simulink model "ATRIAS_vnmc"  (R2015a)
settings: Solver=ode45  StartTime=0.0  StopTime=60  FixedStep=1e-3  MinStep=1e-6  RelTol=1e-3  AbsTol=1e-4
values from neighbouring files (symbols this model uses):
  initial_boom_yaw = initial_boom_yaw + delta_yaw0    [run_model.m]
  max_floor_diff = cost_fun_opts.max_floor_diff    [opt_cmaes.m]    (also in run_model.m; set_all_params_simple.m = 0)
  noise_on_off = cost_fun_opts.noise_on_off    [opt_cmaes.m]    (also in run_model.m; set_all_params_simple.m = 0)
  noise_seed = cost_fun_opts.noise_seed    [opt_cmaes.m]    (also in run_model.m; set_all_params_simple.m = 1)
  noise_variance = cost_fun_opts.noise_variance    [opt_cmaes.m]    (also in run_model.m; set_all_params_simple.m = 0.000174532925199)
  SEA_swing_ctrl_on_off = cost_fun_opts.SEA_swing_ctrl_on_off    [opt_cmaes.m]    (also in run_model.m; set_all_params_simple.m = 0)
  sim_t = simout.twalk    [run_model.m]
  steady_dist = cost_fun_opts.steady_dist    [opt_cmaes.m]    (also in run_model.m; set_all_params_simple.m = 10)
  ts_anim = 0.0333    [run_model.m]
undefined symbols (not defined in the file or in its folder): A1_notch_f1, A2_notch_f1, A_lpf_dtau, A_lpf_velocity, B1_lpf_dtau, B1_lpf_velocity, B1_notch_f1, B2_lpf_dtau, B2_lpf_velocity, B2_notch_f1, b_hmotor, b_leg_spring, b_rotor, base_color_d, boom_color_d, boom_mount_to_center_diagonal, breakaway_friction, c, c_jointstop, com_height_offset, contactThr, coulomb_friction, CtrlPar_theta0, D12_S, D12_T, d_com, ddx_max, ddy_max, delta_phi_max, delta_phi_max_buffer, delta_phi_max_dropoff, delta_phi_min, des_forward_velocity, DS_width, dtau_des_max, dtheta0_vmc, dx0_vmc, dy_max, eref, fblink_color_d, fcut_acceleration, floor_color_d, floor_tile_width, floor_zero_height, FmaxBFSH, FmaxGLU, FmaxHAM, FmaxHFL, FmaxRF, FmaxVAS, FPCtrlPar, friction_linear_zone, g, gain_nodes_sea_torque, gamma_stance_thr, gamma_swing_thr, hip_height, HIP_MTR_MAX_CONT_TORQUE, HIP_MTR_MAX_TORQUE, hshaft_color_d ... (+236)
libraries: sm_lib x280, nesl_utility x174, simulink x114, simulink_extras x58, fl_lib x16, mblibv1 x2, dspswit3 x2
(part 6 of 23)

== system ATRIAS_vnmc/atrias_system/ATRIAS Mechanical System Layer/Torso ==
  COM Sensor : Subsystem
  COM accelerations : Scope
      settings: TimeRange=3  YMin=-750  YMax=2750  SaveName=ScopeData27
  COM dx : Scope
      settings: TimeRange=4  YMin=2.85  YMax=3.95  SaveName=ScopeData24
  COM dy : Scope
      settings: TimeRange=4  YMin=-1.1  YMax=1.2  SaveName=ScopeData32
  COM y pos : Scope
      settings: TimeRange=3  YMin=0.875  YMax=1.375  SaveName=ScopeData23
  CS1 to CS2 : sm_lib/Frames and Transforms/Rigid Transform  TranslationMethod=Cartesian  TranslationLengthUnit=m  TranslationStandardAxis=+Z  TranslationStandardOffset=0  TranslationCartesianOffset=torso_12  TranslationROffset=0  TranslationROffsetUnits=m  TranslationZOffset=0  TranslationZOffsetUnits=m  TranslationThetaOffset=0  TranslationThetaOffsetUnits=deg  RotationMethod=None  RotationAngleUnits=deg  RotationStandardAxis=+Z  RotationAngle=0  RotationArbitraryAxis=[0 0 1]  FollAlignAxisA=+X  BaseAlignAxisA=+Y  FollAlignAxisB=+Y  BaseAlignAxisB=+Z  RotationMatrix=[1 0 0; 0 1 0; 0 0 1]  BlockFunction=simmechanics.library.frames_transforms.rigid_transform
  Frame Data : Subsystem
  Hip Point to COM : sm_lib/Frames and Transforms/Rigid Transform  TranslationMethod=Cartesian  TranslationLengthUnit=m  TranslationStandardAxis=+Z  TranslationStandardOffset=0  TranslationCartesianOffset=[0 d_com 0]  TranslationROffset=0  TranslationROffsetUnits=m  TranslationZOffset=0  TranslationZOffsetUnits=m  TranslationThetaOffset=0  TranslationThetaOffsetUnits=deg  RotationMethod=None  RotationAngleUnits=deg  RotationStandardAxis=+Z  RotationAngle=0  RotationArbitraryAxis=[0 0 1]  FollAlignAxisA=+X  BaseAlignAxisA=+Y  FollAlignAxisB=+Y  BaseAlignAxisB=+Z  RotationMatrix=[1 0 0; 0 1 0; 0 0 1]  BlockFunction=simmechanics.library.frames_transforms.rigid_transform
  Mux : Mux  Inputs=2
  Solid : sm_lib/Body Elements/Solid  InertiaType=Custom  Mass=m_torso  MassUnits=kg  CenterOfMass=com_torso  CenterOfMassUnits=m  MomentsOfInertia=i_torso_moments  MomentsOfInertiaUnits=kg*m^2  ProductsOfInertia=i_torso_products  ProductsOfInertiaUnits=kg*m^2  DensityBased=on  Density=1000  DensityUnits=kg/(m^3)  GraphicType=FromGeometry  MarkerShape=Sphere  MarkerSize=10  MarkerSizeUnits=m  GraphicVisPropType=AdvancedVisualProperties  GraphicDiffuseColor=torso_color_d  GraphicSpecularColor=[0.5 0.5 0.5 1.0]  GraphicAmbientColor=[torso_color_d*0.5 1.0]  GraphicEmissiveColor=[0.0 0.0 0.0 1.0]  GraphicShininess=128  GraphicOpacity=1.0  GeometryShape=FromFile  RectangleSize=[1 1]  RectangleSizeUnits=m  BrickDimensions=[1 1 1]  BrickDimensionUnits=m  CylinderRadius=l_rad  CylinderRadiusUnits=m  CylinderLength=l_seg  CylinderLengthUnits=m  SphereRadius=1  SphereRadiusUnits=m  EllipsoidRadii=[1 1 1]  EllipsoidRadiiUnits=m  ExtrusionCrossSection=[1 1; -1 1; -1 -1; 1 -1]  ExtrusionCrossSectionUnits=m  ExtrusionLength=1  ExtrusionLengthUnits=m  PolygonNumSides=3  PolygonOuterRadius=1  PolygonOuterRadiusUnits=m  ExtGeomFileType=STL  ExtGeomFileName=../0_images/models/torso.STL  ExtGeomFileUnits=m  RevolutionCrossSection=[1 1; 1 -1; 2 -1; 2 1]  RevolutionCrossSectionUnits=m  RevolutionExtent=Full  RevolutionAngle=180  RevolutionAngleUnits=deg  BlockFunction=simmechanics.library.body_elements.solid
  Sum : Sum  Inputs=|++
  Total Energy : Scope
      settings: TimeRange=4  YMin=1080  YMax=1210  SaveName=ScopeData22
  kinetic : Fcn  Expr=0.5*(u(1)^2+u(2)^2)*m_total
  potential : Fcn  Expr=u*m_total*g
  CS1 : PMIOPort  Port=1  Side=Right
  CS2 : PMIOPort  Port=2  Side=Left
  CS3 : PMIOPort  Port=3  Side=Left
  wires:
  COM Sensor/3(dx) -> Mux/1, COM dx/1
  COM Sensor/1(Acceleration) -> COM accelerations/1
  COM Sensor/4(dy) -> COM dy/1, Mux/2
  Mux/1 -> kinetic/1
  COM Sensor/2(y) -> COM y pos/1, potential/1
  kinetic/1 -> Sum/1
  potential/1 -> Sum/2
  Sum/1 -> Total Energy/1
  connections:
  CS1 to CS2/LConn1 -- Frame Data/LConn1 -- CS1/RConn1 -- Solid/RConn1
  CS3/RConn1 -- Hip Point to COM/LConn1 -- CS2/RConn1 -- CS1 to CS2/RConn1
  Hip Point to COM/RConn1 -- COM Sensor/LConn1

== system ATRIAS_vnmc/atrias_system/ATRIAS Mechanical System Layer/Winch ==
  note: Cable cannot push
  Compare To Constant1 : simulink/Logic and Bit Operations/Compare To Constant  relop===  const=-1  OutDataTypeStr=boolean  ZeroCross=off
  Constant1 : Constant  Value=initial_winch_angle
  Constant2 : Constant  Value=0
  Desired Roll Velocity : Constant  Value=0
  Gain2 : Gain  Gain=kp_winch
  Gain3 : Gain  Gain=kd_winch
  PS-Simulink Converter : nesl_utility/PS-Simulink Converter  PhysicalDomain=network_engine_domain  SubClassName=ps_output  LeftPortType=input  RightPortType=output  PseudoPeriodic=off  Frequencies=[]  Unit=1  AffineConversion=off
  PS-Simulink Converter1 : nesl_utility/PS-Simulink Converter  PhysicalDomain=network_engine_domain  SubClassName=ps_output  LeftPortType=input  RightPortType=output  PseudoPeriodic=off  Frequencies=[]  Unit=1  AffineConversion=off
  PS-Simulink Converter2 : nesl_utility/PS-Simulink Converter  PhysicalDomain=network_engine_domain  SubClassName=ps_output  LeftPortType=input  RightPortType=output  PseudoPeriodic=off  Frequencies=[]  Unit=1  AffineConversion=off
  Pitch Frame : sm_lib/Frames and Transforms/Rigid Transform  TranslationMethod=None  TranslationLengthUnit=m  TranslationStandardAxis=+Z  TranslationStandardOffset=0  TranslationCartesianOffset=[0 0 0]  TranslationROffset=0  TranslationROffsetUnits=m  TranslationZOffset=0  TranslationZOffsetUnits=m  TranslationThetaOffset=0  TranslationThetaOffsetUnits=deg  RotationMethod=AlignedAxes  RotationAngleUnits=rad  RotationStandardAxis=+Z  RotationAngle=0  RotationArbitraryAxis=[1 0 0]  FollAlignAxisA=-Z  BaseAlignAxisA=+X  FollAlignAxisB=+Y  BaseAlignAxisB=+Y  RotationMatrix=[1 0 0; 0 1 0; 0 0 1]  BlockFunction=simmechanics.library.frames_transforms.rigid_transform
  Roll Frame : sm_lib/Frames and Transforms/Rigid Transform  TranslationMethod=None  TranslationLengthUnit=m  TranslationStandardAxis=+Z  TranslationStandardOffset=0  TranslationCartesianOffset=[0 0 0]  TranslationROffset=0  TranslationROffsetUnits=m  TranslationZOffset=0  TranslationZOffsetUnits=m  TranslationThetaOffset=0  TranslationThetaOffsetUnits=deg  RotationMethod=AlignedAxes  RotationAngleUnits=rad  RotationStandardAxis=+Z  RotationAngle=0  RotationArbitraryAxis=[1 0 0]  FollAlignAxisA=+X  BaseAlignAxisA=-Z  FollAlignAxisB=+Y  BaseAlignAxisB=+Y  RotationMatrix=[1 0 0; 0 1 0; 0 0 1]  BlockFunction=simmechanics.library.frames_transforms.rigid_transform
  Roll Joint : sm_lib/Joints/Revolute Joint  SenseConstraintForce=off  SenseConstraintForceX=off  SenseConstraintForceY=off  SenseConstraintForceZ=off  SenseConstraintTorque=off  SenseConstraintTorqueX=off  SenseConstraintTorqueY=off  SenseConstraintTorqueZ=off  SenseTotalForce=off  SenseTotalForceX=off  SenseTotalForceY=off  SenseTotalForceZ=off  SenseTotalTorque=off  SenseTotalTorqueX=off  SenseTotalTorqueY=off  SenseTotalTorqueZ=off  CompositeWrenchDir=FollowerOnBase  CompositeWrenchFrame=BaseFrame  EquilibriumPosition=0  EquilibriumPositionUnits=deg  SpringStiffness=0  SpringStiffnessUnits=N*m/deg  DampingCoefficient=0  DampingCoefficientUnits=N*m/(deg/s)  TorqueActuationMode=InputTorque  MotionActuationMode=ComputedMotion  SensePosition=on  SenseVelocity=on  SenseAcceleration=on  SenseTorqueForce=off  PositionTargetSpecify=on  PositionTargetPriority=High  PositionTargetValue=initial_boom_roll  PositionTargetValueUnits=rad  VelocityTargetSpecify=off  VelocityTargetPriority=High  VelocityTargetValue=0  VelocityTargetValueUnits=deg/s  BlockFunction=simmechanics.library.joints.revolute_joint
  Sign1 : Signum  ZeroCross=off
  Simulink-PS Converter : nesl_utility/Simulink-PS Converter  PhysicalDomain=network_engine_domain  SubClassName=ps_input  LeftPortType=input  RightPortType=output  PseudoPeriodic=off  Frequencies=[]  NoiseDistribution=none  NoiseParameters=[]  Unit=1  AffineConversion=off  InputFiltering=off  SimscapeFilterOrder=1  InputFilterTimeConstant=0.001  UdotUserProvided=1
  Sum : Sum  Inputs=+-|
  Sum1 : Sum  Inputs=+|+
  Sum3 : Sum  Inputs=+-|
  Switch : Switch  Threshold=1
  Boom : PMIOPort  Port=1  Side=Right
  Yaw Shaft : PMIOPort  Port=2  Side=Right
  Boom Roll [rad] : Outport
  Boom Roll Velocity [rad/s] : Outport  Port=2
  Boom Roll Acceleration [rad/s^2] : Outport  Port=3
  wires:
  Sum/1 -> Gain2/1
  Sum1/1 -> Switch/3, Sign1/1
  Sign1/1 -> Compare To Constant1/1
  Constant2/1 -> Switch/1
  Compare To Constant1/1 -> Switch/2
  Switch/1 -> Simulink-PS Converter/1
  PS-Simulink Converter/1 -> Sum/2, Boom Roll [rad]/1
  PS-Simulink Converter1/1 -> Boom Roll Velocity [rad/s]/1, Sum3/2
  Desired Roll Velocity/1 -> Sum3/1
  Sum3/1 -> Gain3/1
  Gain2/1 -> Sum1/1
  Gain3/1 -> Sum1/2
  Constant1/1 -> Sum/1
  PS-Simulink Converter2/1 -> Boom Roll Acceleration [rad/s^2]/1
  connections:
  Roll Frame/LConn1 -- Yaw Shaft/RConn1
  Boom/RConn1 -- Pitch Frame/RConn1
  Roll Joint/LConn2 -- Simulink-PS Converter/RConn1
  PS-Simulink Converter/LConn1 -- Roll Joint/RConn2
  PS-Simulink Converter1/LConn1 -- Roll Joint/RConn3
  Roll Joint/LConn1 -- Roll Frame/RConn1
  Roll Joint/RConn1 -- Pitch Frame/LConn1
  Roll Joint/RConn4 -- PS-Simulink Converter2/LConn1

== system ATRIAS_vnmc/atrias_system/ATRIAS Mechanical System Layer/Yaw Joint ==
  PS-Simulink Converter1 : nesl_utility/PS-Simulink Converter  PhysicalDomain=network_engine_domain  SubClassName=ps_output  LeftPortType=input  RightPortType=output  PseudoPeriodic=off  Frequencies=[]  Unit=1  AffineConversion=off
  PS-Simulink Converter2 : nesl_utility/PS-Simulink Converter  PhysicalDomain=network_engine_domain  SubClassName=ps_output  LeftPortType=input  RightPortType=output  PseudoPeriodic=off  Frequencies=[]  Unit=1  AffineConversion=off
  PS-Simulink Converter3 : nesl_utility/PS-Simulink Converter  PhysicalDomain=network_engine_domain  SubClassName=ps_output  LeftPortType=input  RightPortType=output  PseudoPeriodic=off  Frequencies=[]  Unit=1  AffineConversion=off
  Roll Frame : sm_lib/Frames and Transforms/Rigid Transform  TranslationMethod=None  TranslationLengthUnit=m  TranslationStandardAxis=+Z  TranslationStandardOffset=0  TranslationCartesianOffset=[0 0 0]  TranslationROffset=0  TranslationROffsetUnits=m  TranslationZOffset=0  TranslationZOffsetUnits=m  TranslationThetaOffset=0  TranslationThetaOffsetUnits=deg  RotationMethod=AlignedAxes  RotationAngleUnits=rad  RotationStandardAxis=+Z  RotationAngle=0  RotationArbitraryAxis=[1 0 0]  FollAlignAxisA=+Z  BaseAlignAxisA=+Y  FollAlignAxisB=+X  BaseAlignAxisB=+X  RotationMatrix=[1 0 0; 0 1 0; 0 0 1]  BlockFunction=simmechanics.library.frames_transforms.rigid_transform
  Yaw Frame : sm_lib/Frames and Transforms/Rigid Transform  TranslationMethod=None  TranslationLengthUnit=m  TranslationStandardAxis=+Z  TranslationStandardOffset=0  TranslationCartesianOffset=[0 0 0]  TranslationROffset=0  TranslationROffsetUnits=m  TranslationZOffset=0  TranslationZOffsetUnits=m  TranslationThetaOffset=0  TranslationThetaOffsetUnits=deg  RotationMethod=AlignedAxes  RotationAngleUnits=rad  RotationStandardAxis=+Z  RotationAngle=0  RotationArbitraryAxis=[1 0 0]  FollAlignAxisA=+Y  BaseAlignAxisA=+Z  FollAlignAxisB=+X  BaseAlignAxisB=+X  RotationMatrix=[1 0 0; 0 1 0; 0 0 1]  BlockFunction=simmechanics.library.frames_transforms.rigid_transform
  Yaw Joint : sm_lib/Joints/Revolute Joint  SenseConstraintForce=off  SenseConstraintForceX=off  SenseConstraintForceY=off  SenseConstraintForceZ=off  SenseConstraintTorque=off  SenseConstraintTorqueX=off  SenseConstraintTorqueY=off  SenseConstraintTorqueZ=off  SenseTotalForce=off  SenseTotalForceX=off  SenseTotalForceY=off  SenseTotalForceZ=off  SenseTotalTorque=off  SenseTotalTorqueX=off  SenseTotalTorqueY=off  SenseTotalTorqueZ=off  CompositeWrenchDir=FollowerOnBase  CompositeWrenchFrame=BaseFrame  EquilibriumPosition=0  EquilibriumPositionUnits=deg  SpringStiffness=0  SpringStiffnessUnits=N*m/deg  DampingCoefficient=0  DampingCoefficientUnits=N*m/(deg/s)  TorqueActuationMode=NoTorque  MotionActuationMode=ComputedMotion  SensePosition=on  SenseVelocity=on  SenseAcceleration=on  SenseTorqueForce=off  PositionTargetSpecify=on  PositionTargetPriority=High  PositionTargetValue=initial_boom_yaw  PositionTargetValueUnits=rad  VelocityTargetSpecify=on  VelocityTargetPriority=High  VelocityTargetValue=initial_boom_yaw_velocity  VelocityTargetValueUnits=rad/s  BlockFunction=simmechanics.library.joints.revolute_joint
  Yaw Shaft : PMIOPort  Port=1  Side=Right
  Base : PMIOPort  Port=2  Side=Left
  Yaw [rad] : Outport
  Yaw Velocity [rad/s] : Outport  Port=2
  Yaw Acceleration [rad/s^2] : Outport  Port=3
  wires:
  PS-Simulink Converter3/1 -> Yaw [rad]/1
  PS-Simulink Converter1/1 -> Yaw Velocity [rad/s]/1
  PS-Simulink Converter2/1 -> Yaw Acceleration [rad/s^2]/1
  connections:
  Yaw Frame/LConn1 -- Base/RConn1
  Yaw Joint/LConn1 -- Yaw Frame/RConn1
  Roll Frame/LConn1 -- Yaw Joint/RConn1
  Roll Frame/RConn1 -- Yaw Shaft/RConn1
  PS-Simulink Converter3/LConn1 -- Yaw Joint/RConn2
  PS-Simulink Converter1/LConn1 -- Yaw Joint/RConn3
  PS-Simulink Converter2/LConn1 -- Yaw Joint/RConn4

== system ATRIAS_vnmc/atrias_system/ATRIAS Mechanical System Layer/Yaw Shaft ==
  CS1 to CS2 : sm_lib/Frames and Transforms/Rigid Transform  TranslationMethod=Cartesian  TranslationLengthUnit=m  TranslationStandardAxis=+Z  TranslationStandardOffset=0  TranslationCartesianOffset=yshaft_12  TranslationROffset=0  TranslationROffsetUnits=m  TranslationZOffset=0  TranslationZOffsetUnits=m  TranslationThetaOffset=0  TranslationThetaOffsetUnits=deg  RotationMethod=None  RotationAngleUnits=deg  RotationStandardAxis=+Z  RotationAngle=0  RotationArbitraryAxis=[0 0 1]  FollAlignAxisA=+X  BaseAlignAxisA=+Y  FollAlignAxisB=+Y  BaseAlignAxisB=+Z  RotationMatrix=[1 0 0; 0 1 0; 0 0 1]  BlockFunction=simmechanics.library.frames_transforms.rigid_transform
  Frame Data : Subsystem
  Solid : sm_lib/Body Elements/Solid  InertiaType=Custom  Mass=m_yshaft  MassUnits=kg  CenterOfMass=com_yshaft  CenterOfMassUnits=m  MomentsOfInertia=i_yshaft_moments  MomentsOfInertiaUnits=kg*m^2  ProductsOfInertia=i_yshaft_products  ProductsOfInertiaUnits=kg*m^2  DensityBased=on  Density=1000  DensityUnits=kg/(m^3)  GraphicType=FromGeometry  MarkerShape=Sphere  MarkerSize=10  MarkerSizeUnits=m  GraphicVisPropType=AdvancedVisualProperties  GraphicDiffuseColor=yshaft_color_d  GraphicSpecularColor=[0.5 0.5 0.5 1.0]  GraphicAmbientColor=[yshaft_color_d*0.5 1.0]  GraphicEmissiveColor=[0.0 0.0 0.0 1.0]  GraphicShininess=128  GraphicOpacity=1.0  GeometryShape=FromFile  RectangleSize=[1 1]  RectangleSizeUnits=m  BrickDimensions=[1 1 1]  BrickDimensionUnits=m  CylinderRadius=l_rad  CylinderRadiusUnits=m  CylinderLength=l_seg  CylinderLengthUnits=m  SphereRadius=1  SphereRadiusUnits=m  EllipsoidRadii=[1 1 1]  EllipsoidRadiiUnits=m  ExtrusionCrossSection=[1 1; -1 1; -1 -1; 1 -1]  ExtrusionCrossSectionUnits=m  ExtrusionLength=1  ExtrusionLengthUnits=m  PolygonNumSides=3  PolygonOuterRadius=1  PolygonOuterRadiusUnits=m  ExtGeomFileType=STL  ExtGeomFileName=../0_images/models/boom_yaw.stl  ExtGeomFileUnits=m  RevolutionCrossSection=[1 1; 1 -1; 2 -1; 2 1]  RevolutionCrossSectionUnits=m  RevolutionExtent=Full  RevolutionAngle=180  RevolutionAngleUnits=deg  BlockFunction=simmechanics.library.body_elements.solid
  CS1 : PMIOPort  Port=1  Side=Left
  CS2 : PMIOPort  Port=2  Side=Right
  connections:
  CS2/RConn1 -- CS1 to CS2/RConn1
  CS1/RConn1 -- CS1 to CS2/LConn1 -- Solid/RConn1 -- Frame Data/LConn1

== system ATRIAS_vnmc/atrias_system/ATRIAS Mechanical System Layer/gamma min//max visualization ==
  Center-to-Hip{,1..3} (4 alike) : sm_lib/Frames and Transforms/Rigid Transform  TranslationMethod=Cartesian  TranslationLengthUnit=m  TranslationStandardAxis=+Z  TranslationStandardOffset=0  TranslationCartesianOffset=[-D12_T 0 0]  TranslationROffset=0  TranslationROffsetUnits=m  TranslationZOffset=0  TranslationZOffsetUnits=m  TranslationThetaOffset=0  TranslationThetaOffsetUnits=deg  RotationMethod=None  RotationAngleUnits=deg  RotationStandardAxis=+Z  RotationAngle=0  RotationArbitraryAxis=[0 0 1]  FollAlignAxisA=+X  BaseAlignAxisA=+Y  FollAlignAxisB=+Y  BaseAlignAxisB=+Z  RotationMatrix=[1 0 0; 0 1 0; 0 0 1]  BlockFunction=simmechanics.library.frames_transforms.rigid_transform
  Constant : Constant  Value=gamma_swing_thr
  Constant1 : Constant  Value=gamma_stance_thr
  Constant2 : Constant  Value=2*pi-gamma_swing_thr
  Constant3 : Constant  Value=2*pi-gamma_stance_thr
  Gamma visualization : sm_lib/Body Elements/Solid  InertiaType=PointMass  Mass=0  MassUnits=kg  CenterOfMass=[0 0 0]  CenterOfMassUnits=m  MomentsOfInertia=[1 1 1]  MomentsOfInertiaUnits=kg*m^2  ProductsOfInertia=[0 0 0]  ProductsOfInertiaUnits=kg*m^2  DensityBased=on  Density=1000  DensityUnits=kg/(m^3)  GraphicType=FromGeometry  MarkerShape=Sphere  MarkerSize=10  MarkerSizeUnits=m  GraphicVisPropType=SimpleVisualProperties  GraphicDiffuseColor=[0.4 1.0 1.0]  GraphicSpecularColor=[0.5 0.5 0.5 1.0]  GraphicAmbientColor=[0.15 0.15 0.15 1.0]  GraphicEmissiveColor=[0.0 0.0 0.0 1.0]  GraphicShininess=75  GraphicOpacity=0.75  GeometryShape=Brick  RectangleSize=[1 1]  RectangleSizeUnits=m  BrickDimensions=[leg_length_max 0.015 0.05]  BrickDimensionUnits=m  CylinderRadius=1  CylinderRadiusUnits=m  CylinderLength=1  CylinderLengthUnits=m  SphereRadius=1  SphereRadiusUnits=m  EllipsoidRadii=[1 1 1]  EllipsoidRadiiUnits=m  ExtrusionCrossSection=[1 1; -1 1; -1 -1; 1 -1]  ExtrusionCrossSectionUnits=m  ExtrusionLength=1  ExtrusionLengthUnits=m  PolygonNumSides=3  PolygonOuterRadius=1  PolygonOuterRadiusUnits=m  ExtGeomFileType=STL  ExtGeomFileUnits=m  RevolutionCrossSection=[1 1; 1 -1; 2 -1; 2 1]  RevolutionCrossSectionUnits=m  RevolutionExtent=Full  RevolutionAngle=180  RevolutionAngleUnits=deg  BlockFunction=simmechanics.library.body_elements.solid
  Gamma visualization1 : sm_lib/Body Elements/Solid  InertiaType=PointMass  Mass=0  MassUnits=kg  CenterOfMass=[0 0 0]  CenterOfMassUnits=m  MomentsOfInertia=[1 1 1]  MomentsOfInertiaUnits=kg*m^2  ProductsOfInertia=[0 0 0]  ProductsOfInertiaUnits=kg*m^2  DensityBased=on  Density=1000  DensityUnits=kg/(m^3)  GraphicType=FromGeometry  MarkerShape=Sphere  MarkerSize=10  MarkerSizeUnits=m  GraphicVisPropType=SimpleVisualProperties  GraphicDiffuseColor=[0.4 1.0 1.0]  GraphicSpecularColor=[0.5 0.5 0.5 1.0]  GraphicAmbientColor=[0.15 0.15 0.15 1.0]  GraphicEmissiveColor=[0.0 0.0 0.0 1.0]  GraphicShininess=75  GraphicOpacity=0.75  GeometryShape=Brick  RectangleSize=[1 1]  RectangleSizeUnits=m  BrickDimensions=[leg_length_min 0.015 0.05]  BrickDimensionUnits=m  CylinderRadius=1  CylinderRadiusUnits=m  CylinderLength=1  CylinderLengthUnits=m  SphereRadius=1  SphereRadiusUnits=m  EllipsoidRadii=[1 1 1]  EllipsoidRadiiUnits=m  ExtrusionCrossSection=[1 1; -1 1; -1 -1; 1 -1]  ExtrusionCrossSectionUnits=m  ExtrusionLength=1  ExtrusionLengthUnits=m  PolygonNumSides=3  PolygonOuterRadius=1  PolygonOuterRadiusUnits=m  ExtGeomFileType=STL  ExtGeomFileUnits=m  RevolutionCrossSection=[1 1; 1 -1; 2 -1; 2 1]  RevolutionCrossSectionUnits=m  RevolutionExtent=Full  RevolutionAngle=180  RevolutionAngleUnits=deg  BlockFunction=simmechanics.library.body_elements.solid
  Gamma visualization2 : sm_lib/Body Elements/Solid  InertiaType=PointMass  Mass=0  MassUnits=kg  CenterOfMass=[0 0 0]  CenterOfMassUnits=m  MomentsOfInertia=[1 1 1]  MomentsOfInertiaUnits=kg*m^2  ProductsOfInertia=[0 0 0]  ProductsOfInertiaUnits=kg*m^2  DensityBased=on  Density=1000  DensityUnits=kg/(m^3)  GraphicType=FromGeometry  MarkerShape=Sphere  MarkerSize=10  MarkerSizeUnits=m  GraphicVisPropType=SimpleVisualProperties  GraphicDiffuseColor=[1.0 0.6 0.4]  GraphicSpecularColor=[0.5 0.5 0.5 1.0]  GraphicAmbientColor=[0.15 0.15 0.15 1.0]  GraphicEmissiveColor=[0.0 0.0 0.0 1.0]  GraphicShininess=75  GraphicOpacity=0.75  GeometryShape=Brick  RectangleSize=[1 1]  RectangleSizeUnits=m  BrickDimensions=[leg_length_max 0.015 0.05]  BrickDimensionUnits=m  CylinderRadius=1  CylinderRadiusUnits=m  CylinderLength=1  CylinderLengthUnits=m  SphereRadius=1  SphereRadiusUnits=m  EllipsoidRadii=[1 1 1]  EllipsoidRadiiUnits=m  ExtrusionCrossSection=[1 1; -1 1; -1 -1; 1 -1]  ExtrusionCrossSectionUnits=m  ExtrusionLength=1  ExtrusionLengthUnits=m  PolygonNumSides=3  PolygonOuterRadius=1  PolygonOuterRadiusUnits=m  ExtGeomFileType=STL  ExtGeomFileUnits=m  RevolutionCrossSection=[1 1; 1 -1; 2 -1; 2 1]  RevolutionCrossSectionUnits=m  RevolutionExtent=Full  RevolutionAngle=180  RevolutionAngleUnits=deg  BlockFunction=simmechanics.library.body_elements.solid
  Gamma visualization3 : sm_lib/Body Elements/Solid  InertiaType=PointMass  Mass=0  MassUnits=kg  CenterOfMass=[0 0 0]  CenterOfMassUnits=m  MomentsOfInertia=[1 1 1]  MomentsOfInertiaUnits=kg*m^2  ProductsOfInertia=[0 0 0]  ProductsOfInertiaUnits=kg*m^2  DensityBased=on  Density=1000  DensityUnits=kg/(m^3)  GraphicType=FromGeometry  MarkerShape=Sphere  MarkerSize=10  MarkerSizeUnits=m  GraphicVisPropType=SimpleVisualProperties  GraphicDiffuseColor=[1.0 0.6 0.4]  GraphicSpecularColor=[0.5 0.5 0.5 1.0]  GraphicAmbientColor=[0.15 0.15 0.15 1.0]  GraphicEmissiveColor=[0.0 0.0 0.0 1.0]  GraphicShininess=75  GraphicOpacity=0.75  GeometryShape=Brick  RectangleSize=[1 1]  RectangleSizeUnits=m  BrickDimensions=[leg_length_min 0.015 0.05]  BrickDimensionUnits=m  CylinderRadius=1  CylinderRadiusUnits=m  CylinderLength=1  CylinderLengthUnits=m  SphereRadius=1  SphereRadiusUnits=m  EllipsoidRadii=[1 1 1]  EllipsoidRadiiUnits=m  ExtrusionCrossSection=[1 1; -1 1; -1 -1; 1 -1]  ExtrusionCrossSectionUnits=m  ExtrusionLength=1  ExtrusionLengthUnits=m  PolygonNumSides=3  PolygonOuterRadius=1  PolygonOuterRadiusUnits=m  ExtGeomFileType=STL  ExtGeomFileUnits=m  RevolutionCrossSection=[1 1; 1 -1; 2 -1; 2 1]  RevolutionCrossSectionUnits=m  RevolutionExtent=Full  RevolutionAngle=180  RevolutionAngleUnits=deg  BlockFunction=simmechanics.library.body_elements.solid
  Memory{,1..3} (4 alike) : Memory
  Revolute Joint{,1..3} (4 alike) : sm_lib/Joints/Revolute Joint  SenseConstraintForce=off  SenseConstraintForceX=off  SenseConstraintForceY=off  SenseConstraintForceZ=off  SenseConstraintTorque=off  SenseConstraintTorqueX=off  SenseConstraintTorqueY=off  SenseConstraintTorqueZ=off  SenseTotalForce=off  SenseTotalForceX=off  SenseTotalForceY=off  SenseTotalForceZ=off  SenseTotalTorque=off  SenseTotalTorqueX=off  SenseTotalTorqueY=off  SenseTotalTorqueZ=off  CompositeWrenchDir=FollowerOnBase  CompositeWrenchFrame=BaseFrame  EquilibriumPosition=0  EquilibriumPositionUnits=deg  SpringStiffness=0  SpringStiffnessUnits=N*m/deg  DampingCoefficient=0  DampingCoefficientUnits=N*m/(deg/s)  TorqueActuationMode=ComputedTorque  MotionActuationMode=InputMotion  SensePosition=off  SenseVelocity=off  SenseAcceleration=off  SenseTorqueForce=off  PositionTargetSpecify=on  PositionTargetPriority=High  PositionTargetValue=Lv230  PositionTargetValueUnits=rad  VelocityTargetSpecify=off  VelocityTargetPriority=High  VelocityTargetValue=0  VelocityTargetValueUnits=rad/s  BlockFunction=simmechanics.library.joints.revolute_joint
  Rotate 90deg{,1..3} (4 alike) : sm_lib/Frames and Transforms/Rigid Transform  TranslationMethod=Cartesian  TranslationLengthUnit=m  TranslationStandardAxis=+Z  TranslationStandardOffset=0  TranslationCartesianOffset=[0,0,0]  TranslationROffset=0  TranslationROffsetUnits=m  TranslationZOffset=0  TranslationZOffsetUnits=m  TranslationThetaOffset=0  TranslationThetaOffsetUnits=deg  RotationMethod=StandardAxis  RotationAngleUnits=deg  RotationStandardAxis=+Z  RotationAngle=90  RotationArbitraryAxis=[0 0 1]  FollAlignAxisA=+X  BaseAlignAxisA=+Y  FollAlignAxisB=+Y  BaseAlignAxisB=+Z  RotationMatrix=[1 0 0; 0 1 0; 0 0 1]  BlockFunction=simmechanics.library.frames_transforms.rigid_transform
  Simulink-PS Converter{,1..3} (4 alike) : nesl_utility/Simulink-PS Converter  PhysicalDomain=network_engine_domain  SubClassName=ps_input  LeftPortType=input  RightPortType=output  PseudoPeriodic=off  Frequencies=[]  NoiseDistribution=none  NoiseParameters=[]  Unit=1  AffineConversion=off  InputFiltering=on  SimscapeFilterOrder=2  InputFilterTimeConstant=sample_time  UdotUserProvided=1
  Sum{,1..3} (4 alike) : Sum  Inputs=|+-
  Hip : PMIOPort  Port=1  Side=Right
  wires:
  Constant/1 -> Sum/1
  Memory/1 -> Simulink-PS Converter/1
  Sum/1 -> Memory/1
  [theta] -> Sum/2
  Constant1/1 -> Sum1/1
  Memory1/1 -> Simulink-PS Converter1/1
  Sum1/1 -> Memory1/1
  [theta] -> Sum1/2
  Constant2/1 -> Sum2/1
  Memory2/1 -> Simulink-PS Converter2/1
  Sum2/1 -> Memory2/1
  [theta] -> Sum2/2
  Constant3/1 -> Sum3/1
  Memory3/1 -> Simulink-PS Converter3/1
  Sum3/1 -> Memory3/1
  [theta] -> Sum3/2
  connections:
  Center-to-Hip/LConn1 -- Gamma visualization/RConn1
  Revolute Joint/RConn1 -- Rotate 90deg/RConn1
  Simulink-PS Converter/RConn1 -- Revolute Joint/LConn2
  Center-to-Hip/RConn1 -- Revolute Joint/LConn1
  Rotate 90deg2/LConn1 -- Hip/RConn1 -- Rotate 90deg1/LConn1 -- Rotate 90deg/LConn1 -- Rotate 90deg3/LConn1
  Center-to-Hip1/RConn1 -- Revolute Joint1/LConn1
  Simulink-PS Converter1/RConn1 -- Revolute Joint1/LConn2
  Revolute Joint1/RConn1 -- Rotate 90deg1/RConn1
  Center-to-Hip1/LConn1 -- Gamma visualization1/RConn1
  Center-to-Hip3/LConn1 -- Gamma visualization3/RConn1
  Center-to-Hip2/LConn1 -- Gamma visualization2/RConn1
  Simulink-PS Converter3/RConn1 -- Revolute Joint3/LConn2
  Simulink-PS Converter2/RConn1 -- Revolute Joint2/LConn2
  Revolute Joint2/RConn1 -- Rotate 90deg2/RConn1
  Revolute Joint3/RConn1 -- Rotate 90deg3/RConn1
  Center-to-Hip2/RConn1 -- Revolute Joint2/LConn1
  Center-to-Hip3/RConn1 -- Revolute Joint3/LConn1

== system ATRIAS_vnmc/atrias_system/ATRIAS Mechanical System Layer/gamma min//max visualization1 ==
  Center-to-Hip{,1..3} (4 alike) : sm_lib/Frames and Transforms/Rigid Transform  TranslationMethod=Cartesian  TranslationLengthUnit=m  TranslationStandardAxis=+Z  TranslationStandardOffset=0  TranslationCartesianOffset=[-D12_T 0 0]  TranslationROffset=0  TranslationROffsetUnits=m  TranslationZOffset=0  TranslationZOffsetUnits=m  TranslationThetaOffset=0  TranslationThetaOffsetUnits=deg  RotationMethod=None  RotationAngleUnits=deg  RotationStandardAxis=+Z  RotationAngle=0  RotationArbitraryAxis=[0 0 1]  FollAlignAxisA=+X  BaseAlignAxisA=+Y  FollAlignAxisB=+Y  BaseAlignAxisB=+Z  RotationMatrix=[1 0 0; 0 1 0; 0 0 1]  BlockFunction=simmechanics.library.frames_transforms.rigid_transform
  Constant : Constant  Value=gamma_swing_thr
  Constant1 : Constant  Value=gamma_stance_thr
  Constant2 : Constant  Value=2*pi-gamma_swing_thr
  Constant3 : Constant  Value=2*pi-gamma_stance_thr
  Gamma visualization : sm_lib/Body Elements/Solid  InertiaType=PointMass  Mass=0  MassUnits=kg  CenterOfMass=[0 0 0]  CenterOfMassUnits=m  MomentsOfInertia=[1 1 1]  MomentsOfInertiaUnits=kg*m^2  ProductsOfInertia=[0 0 0]  ProductsOfInertiaUnits=kg*m^2  DensityBased=on  Density=1000  DensityUnits=kg/(m^3)  GraphicType=FromGeometry  MarkerShape=Sphere  MarkerSize=10  MarkerSizeUnits=m  GraphicVisPropType=SimpleVisualProperties  GraphicDiffuseColor=[0.4 1.0 1.0]  GraphicSpecularColor=[0.5 0.5 0.5 1.0]  GraphicAmbientColor=[0.15 0.15 0.15 1.0]  GraphicEmissiveColor=[0.0 0.0 0.0 1.0]  GraphicShininess=75  GraphicOpacity=0.75  GeometryShape=Brick  RectangleSize=[1 1]  RectangleSizeUnits=m  BrickDimensions=[leg_length_max 0.015 0.05]  BrickDimensionUnits=m  CylinderRadius=1  CylinderRadiusUnits=m  CylinderLength=1  CylinderLengthUnits=m  SphereRadius=1  SphereRadiusUnits=m  EllipsoidRadii=[1 1 1]  EllipsoidRadiiUnits=m  ExtrusionCrossSection=[1 1; -1 1; -1 -1; 1 -1]  ExtrusionCrossSectionUnits=m  ExtrusionLength=1  ExtrusionLengthUnits=m  PolygonNumSides=3  PolygonOuterRadius=1  PolygonOuterRadiusUnits=m  ExtGeomFileType=STL  ExtGeomFileUnits=m  RevolutionCrossSection=[1 1; 1 -1; 2 -1; 2 1]  RevolutionCrossSectionUnits=m  RevolutionExtent=Full  RevolutionAngle=180  RevolutionAngleUnits=deg  BlockFunction=simmechanics.library.body_elements.solid
  Gamma visualization1 : sm_lib/Body Elements/Solid  InertiaType=PointMass  Mass=0  MassUnits=kg  CenterOfMass=[0 0 0]  CenterOfMassUnits=m  MomentsOfInertia=[1 1 1]  MomentsOfInertiaUnits=kg*m^2  ProductsOfInertia=[0 0 0]  ProductsOfInertiaUnits=kg*m^2  DensityBased=on  Density=1000  DensityUnits=kg/(m^3)  GraphicType=FromGeometry  MarkerShape=Sphere  MarkerSize=10  MarkerSizeUnits=m  GraphicVisPropType=SimpleVisualProperties  GraphicDiffuseColor=[0.4 1.0 1.0]  GraphicSpecularColor=[0.5 0.5 0.5 1.0]  GraphicAmbientColor=[0.15 0.15 0.15 1.0]  GraphicEmissiveColor=[0.0 0.0 0.0 1.0]  GraphicShininess=75  GraphicOpacity=0.75  GeometryShape=Brick  RectangleSize=[1 1]  RectangleSizeUnits=m  BrickDimensions=[leg_length_min 0.015 0.05]  BrickDimensionUnits=m  CylinderRadius=1  CylinderRadiusUnits=m  CylinderLength=1  CylinderLengthUnits=m  SphereRadius=1  SphereRadiusUnits=m  EllipsoidRadii=[1 1 1]  EllipsoidRadiiUnits=m  ExtrusionCrossSection=[1 1; -1 1; -1 -1; 1 -1]  ExtrusionCrossSectionUnits=m  ExtrusionLength=1  ExtrusionLengthUnits=m  PolygonNumSides=3  PolygonOuterRadius=1  PolygonOuterRadiusUnits=m  ExtGeomFileType=STL  ExtGeomFileUnits=m  RevolutionCrossSection=[1 1; 1 -1; 2 -1; 2 1]  RevolutionCrossSectionUnits=m  RevolutionExtent=Full  RevolutionAngle=180  RevolutionAngleUnits=deg  BlockFunction=simmechanics.library.body_elements.solid
  Gamma visualization2 : sm_lib/Body Elements/Solid  InertiaType=PointMass  Mass=0  MassUnits=kg  CenterOfMass=[0 0 0]  CenterOfMassUnits=m  MomentsOfInertia=[1 1 1]  MomentsOfInertiaUnits=kg*m^2  ProductsOfInertia=[0 0 0]  ProductsOfInertiaUnits=kg*m^2  DensityBased=on  Density=1000  DensityUnits=kg/(m^3)  GraphicType=FromGeometry  MarkerShape=Sphere  MarkerSize=10  MarkerSizeUnits=m  GraphicVisPropType=SimpleVisualProperties  GraphicDiffuseColor=[1.0 0.6 0.4]  GraphicSpecularColor=[0.5 0.5 0.5 1.0]  GraphicAmbientColor=[0.15 0.15 0.15 1.0]  GraphicEmissiveColor=[0.0 0.0 0.0 1.0]  GraphicShininess=75  GraphicOpacity=0.75  GeometryShape=Brick  RectangleSize=[1 1]  RectangleSizeUnits=m  BrickDimensions=[leg_length_max 0.015 0.05]  BrickDimensionUnits=m  CylinderRadius=1  CylinderRadiusUnits=m  CylinderLength=1  CylinderLengthUnits=m  SphereRadius=1  SphereRadiusUnits=m  EllipsoidRadii=[1 1 1]  EllipsoidRadiiUnits=m  ExtrusionCrossSection=[1 1; -1 1; -1 -1; 1 -1]  ExtrusionCrossSectionUnits=m  ExtrusionLength=1  ExtrusionLengthUnits=m  PolygonNumSides=3  PolygonOuterRadius=1  PolygonOuterRadiusUnits=m  ExtGeomFileType=STL  ExtGeomFileUnits=m  RevolutionCrossSection=[1 1; 1 -1; 2 -1; 2 1]  RevolutionCrossSectionUnits=m  RevolutionExtent=Full  RevolutionAngle=180  RevolutionAngleUnits=deg  BlockFunction=simmechanics.library.body_elements.solid
  Gamma visualization3 : sm_lib/Body Elements/Solid  InertiaType=PointMass  Mass=0  MassUnits=kg  CenterOfMass=[0 0 0]  CenterOfMassUnits=m  MomentsOfInertia=[1 1 1]  MomentsOfInertiaUnits=kg*m^2  ProductsOfInertia=[0 0 0]  ProductsOfInertiaUnits=kg*m^2  DensityBased=on  Density=1000  DensityUnits=kg/(m^3)  GraphicType=FromGeometry  MarkerShape=Sphere  MarkerSize=10  MarkerSizeUnits=m  GraphicVisPropType=SimpleVisualProperties  GraphicDiffuseColor=[1.0 0.6 0.4]  GraphicSpecularColor=[0.5 0.5 0.5 1.0]  GraphicAmbientColor=[0.15 0.15 0.15 1.0]  GraphicEmissiveColor=[0.0 0.0 0.0 1.0]  GraphicShininess=75  GraphicOpacity=0.75  GeometryShape=Brick  RectangleSize=[1 1]  RectangleSizeUnits=m  BrickDimensions=[leg_length_min 0.015 0.05]  BrickDimensionUnits=m  CylinderRadius=1  CylinderRadiusUnits=m  CylinderLength=1  CylinderLengthUnits=m  SphereRadius=1  SphereRadiusUnits=m  EllipsoidRadii=[1 1 1]  EllipsoidRadiiUnits=m  ExtrusionCrossSection=[1 1; -1 1; -1 -1; 1 -1]  ExtrusionCrossSectionUnits=m  ExtrusionLength=1  ExtrusionLengthUnits=m  PolygonNumSides=3  PolygonOuterRadius=1  PolygonOuterRadiusUnits=m  ExtGeomFileType=STL  ExtGeomFileUnits=m  RevolutionCrossSection=[1 1; 1 -1; 2 -1; 2 1]  RevolutionCrossSectionUnits=m  RevolutionExtent=Full  RevolutionAngle=180  RevolutionAngleUnits=deg  BlockFunction=simmechanics.library.body_elements.solid
  Memory{,1..3} (4 alike) : Memory
  Revolute Joint{,1..3} (4 alike) : sm_lib/Joints/Revolute Joint  SenseConstraintForce=off  SenseConstraintForceX=off  SenseConstraintForceY=off  SenseConstraintForceZ=off  SenseConstraintTorque=off  SenseConstraintTorqueX=off  SenseConstraintTorqueY=off  SenseConstraintTorqueZ=off  SenseTotalForce=off  SenseTotalForceX=off  SenseTotalForceY=off  SenseTotalForceZ=off  SenseTotalTorque=off  SenseTotalTorqueX=off  SenseTotalTorqueY=off  SenseTotalTorqueZ=off  CompositeWrenchDir=FollowerOnBase  CompositeWrenchFrame=BaseFrame  EquilibriumPosition=0  EquilibriumPositionUnits=deg  SpringStiffness=0  SpringStiffnessUnits=N*m/deg  DampingCoefficient=0  DampingCoefficientUnits=N*m/(deg/s)  TorqueActuationMode=ComputedTorque  MotionActuationMode=InputMotion  SensePosition=off  SenseVelocity=off  SenseAcceleration=off  SenseTorqueForce=off  PositionTargetSpecify=on  PositionTargetPriority=High  PositionTargetValue=Lv230  PositionTargetValueUnits=rad  VelocityTargetSpecify=off  VelocityTargetPriority=High  VelocityTargetValue=0  VelocityTargetValueUnits=rad/s  BlockFunction=simmechanics.library.joints.revolute_joint
  Rotate 90deg{,1..3} (4 alike) : sm_lib/Frames and Transforms/Rigid Transform  TranslationMethod=Cartesian  TranslationLengthUnit=m  TranslationStandardAxis=+Z  TranslationStandardOffset=0  TranslationCartesianOffset=[0,0,0]  TranslationROffset=0  TranslationROffsetUnits=m  TranslationZOffset=0  TranslationZOffsetUnits=m  TranslationThetaOffset=0  TranslationThetaOffsetUnits=deg  RotationMethod=StandardAxis  RotationAngleUnits=deg  RotationStandardAxis=+Z  RotationAngle=90  RotationArbitraryAxis=[0 0 1]  FollAlignAxisA=+X  BaseAlignAxisA=+Y  FollAlignAxisB=+Y  BaseAlignAxisB=+Z  RotationMatrix=[1 0 0; 0 1 0; 0 0 1]  BlockFunction=simmechanics.library.frames_transforms.rigid_transform
  Simulink-PS Converter{,1..3} (4 alike) : nesl_utility/Simulink-PS Converter  PhysicalDomain=network_engine_domain  SubClassName=ps_input  LeftPortType=input  RightPortType=output  PseudoPeriodic=off  Frequencies=[]  NoiseDistribution=none  NoiseParameters=[]  Unit=1  AffineConversion=off  InputFiltering=on  SimscapeFilterOrder=2  InputFilterTimeConstant=sample_time  UdotUserProvided=1
  Sum{,1..3} (4 alike) : Sum  Inputs=|+-
  Hip : PMIOPort  Port=1  Side=Right
  wires:
  [theta] -> Sum3/2
  Sum3/1 -> Memory3/1
  Memory3/1 -> Simulink-PS Converter3/1
  Constant3/1 -> Sum3/1
  [theta] -> Sum2/2
  Sum2/1 -> Memory2/1
  Memory2/1 -> Simulink-PS Converter2/1
  Constant2/1 -> Sum2/1
  [theta] -> Sum1/2
  Sum1/1 -> Memory1/1
  Memory1/1 -> Simulink-PS Converter1/1
  Constant1/1 -> Sum1/1
  [theta] -> Sum/2
  Sum/1 -> Memory/1
  Memory/1 -> Simulink-PS Converter/1
  Constant/1 -> Sum/1
  connections:
  Center-to-Hip3/RConn1 -- Revolute Joint3/LConn1
  Center-to-Hip2/RConn1 -- Revolute Joint2/LConn1
  Revolute Joint3/RConn1 -- Rotate 90deg3/RConn1
  Revolute Joint2/RConn1 -- Rotate 90deg2/RConn1
  Simulink-PS Converter2/RConn1 -- Revolute Joint2/LConn2
  Simulink-PS Converter3/RConn1 -- Revolute Joint3/LConn2
  Center-to-Hip2/LConn1 -- Gamma visualization2/RConn1
  Center-to-Hip3/LConn1 -- Gamma visualization3/RConn1
  Center-to-Hip1/LConn1 -- Gamma visualization1/RConn1
  Revolute Joint1/RConn1 -- Rotate 90deg1/RConn1
  Simulink-PS Converter1/RConn1 -- Revolute Joint1/LConn2
  Center-to-Hip1/RConn1 -- Revolute Joint1/LConn1
  Rotate 90deg2/LConn1 -- Rotate 90deg3/LConn1 -- Rotate 90deg/LConn1 -- Rotate 90deg1/LConn1 -- Hip/RConn1
  Center-to-Hip/RConn1 -- Revolute Joint/LConn1
  Simulink-PS Converter/RConn1 -- Revolute Joint/LConn2
  Revolute Joint/RConn1 -- Rotate 90deg/RConn1
  Center-to-Hip/LConn1 -- Gamma visualization/RConn1

== system ATRIAS_vnmc/atrias_system/Discretize Sensors, Add Noise/Low Pass Discrete Derivative f(sample_time, A_lpf_velocity, B1_lpf_velocity, B2_lpf_velocity) ==
  q : Inport
  Gain1 : Gain  Gain=1/sample_time
  discrete difference : Subsystem
  two_pole_filter : DiscreteTransferFcn  Numerator=[A_lpf_velocity 0 0]  Denominator=[1 B1_lpf_velocity B2_lpf_velocity]  SampleTime=sample_time
  dq : Outport
  wires:
  q/1 -> discrete difference/1(x)
  two_pole_filter/1 -> dq/1
  Gain1/1 -> two_pole_filter/1
  discrete difference/1(dx) -> Gain1/1

== system ATRIAS_vnmc/atrias_system/Discretize Sensors, Add Noise/scale by noise_variance, saturate by [-3*noise_variance,3*noise_variance] ==
  Variance = 1 : Inport
  Enable : EnablePort  StatesWhenEnabling=reset
  Gain : Gain  Gain=noise_variance
  "[-3*noise_variance,3*noise_variance]" : Saturate  UpperLimit=3*noise_variance  LowerLimit=-3*noise_variance
  Variance = noise_variance : Outport  InitialOutput=0
  wires:
  Variance = 1/1 -> Gain/1
  Gain/1 -> "[-3*noise_variance,3*noise_variance]"/1
  "[-3*noise_variance,3*noise_variance]"/1 -> Variance = noise_variance/1

== system ATRIAS_vnmc/atrias_system/Ground Contact/L Contact ==
  note: 3D Ground Interaction Model
  Env : Inport
  3D Contact : Subsystem
  Demux2 : Demux  Outputs=[1 3 3]
  External Force and Torque : sm_lib/Forces and Torques/External Force and Torque  ForceResolutionFrame=World  EnableForceX=off  EnableForceY=off  EnableForceZ=off  EnableForce=on  TorqueResolutionFrame=AttachedFrame  EnableTorqueX=off  EnableTorqueY=off  EnableTorqueZ=off  EnableTorque=off  BlockFunction=simmechanics.library.forces_torques.external_force_torque
  Mux1 : Mux  Inputs=3
  Mux2 : Mux  Inputs=3
  PS-Simulink Converter{1..6} (6 alike) : nesl_utility/PS-Simulink Converter  PhysicalDomain=network_engine_domain  SubClassName=ps_output  LeftPortType=input  RightPortType=output  PseudoPeriodic=off  Frequencies=[]  Unit=1  AffineConversion=off
  Simulink-PS Converter : nesl_utility/Simulink-PS Converter  PhysicalDomain=network_engine_domain  SubClassName=ps_input  LeftPortType=input  RightPortType=output  PseudoPeriodic=off  Frequencies=[]  NoiseDistribution=none  NoiseParameters=[]  Unit=1  AffineConversion=off  InputFiltering=off  SimscapeFilterOrder=1  InputFilterTimeConstant=0.001  UdotUserProvided=1
  Sum : Sum  Inputs=|+-
  Sum1 : Sum
  Transform Sensor : sm_lib/Frames and Transforms/Transform Sensor  MeasurementFrame=World  SenseAngle=off  SenseAxis=off  SenseAngle1=off  SenseAngle2=off  SenseAngle3=off  SenseQ=off  SenseR=off  SenseOmegaX=off  SenseOmegaY=off  SenseOmegaZ=off  SenseOmega1=off  SenseOmega2=off  SenseOmega3=off  SenseQDot=off  SenseRDot=off  SenseAlphaX=off  SenseAlphaY=off  SenseAlphaZ=off  SenseAlpha1=off  SenseAlpha2=off  SenseAlpha3=off  SenseQDDot=off  SenseRDDot=off  SenseX=on  SenseY=on  SenseZ=on  SenseRad=off  SenseAzim=off  SenseDist=off  SenseInc=off  SenseXDot=on  SenseYDot=on  SenseZDot=on  SenseRadDot=off  SenseAzimDot=off  SenseDistDot=off  SenseIncDot=off  SenseXDDot=off  SenseYDDot=off  SenseZDDot=off  SenseRadDDot=off  SenseAzimDDot=off  SenseDistDDot=off  SenseIncDDot=off  BlockFunction=simmechanics.library.frames_transforms.transform_sensor
  World Frame : sm_lib/Frames and Transforms/World Frame  BlockFunction=simmechanics.library.frames_transforms.world_frame
  contact? : simulink/Logic and Bit Operations/Compare To Zero  relop=<=  OutDataTypeStr=boolean
  y : Selector  InputPortWidth=3  Indices=2
  F : PMIOPort  Port=1  Side=Left
  RBallCnt : Outport
  GRF [N N N] : Outport  Port=2
  xyzFoot : Outport  Port=3
  wires:
  contact?/1 -> 3D Contact/Enable, RBallCnt/1  "cnt"
  Mux1/1 -> xyzFoot/1, 3D Contact/3(pVec [m m m]), y/1  "pos"
  Mux2/1 -> 3D Contact/4(vVec [m/s m/s m/s])
  Env/1 -> Demux2/1
  3D Contact/1(FnVec [N N N]) -> Sum1/1
  3D Contact/2(FtVec [N N N]) -> Sum1/2
  Sum1/1 -> Simulink-PS Converter/1, GRF [N N N]/1
  Sum/1 -> contact?/1
  y/1 -> Sum/1
  Demux2/1 -> Sum/2  "EnvHeight"
  Demux2/3 -> 3D Contact/2(nVec [m m m])  "Normal Vector nVec"
  Demux2/2 -> 3D Contact/1(RefPt [m m m])  "Reference Point RefPt"
  PS-Simulink Converter2/1 -> Mux1/1
  PS-Simulink Converter1/1 -> Mux1/2
  PS-Simulink Converter3/1 -> Mux1/3
  PS-Simulink Converter5/1 -> Mux2/1
  PS-Simulink Converter4/1 -> Mux2/2
  PS-Simulink Converter6/1 -> Mux2/3
  connections:
  External Force and Torque/LConn1 -- Simulink-PS Converter/RConn1
  F/RConn1 -- Transform Sensor/RConn1 -- External Force and Torque/RConn1
  World Frame/RConn1 -- Transform Sensor/LConn1
  PS-Simulink Converter2/LConn1 -- Transform Sensor/RConn2
  Transform Sensor/RConn3 -- PS-Simulink Converter1/LConn1
  Transform Sensor/RConn4 -- PS-Simulink Converter3/LConn1
  Transform Sensor/RConn5 -- PS-Simulink Converter5/LConn1
  Transform Sensor/RConn7 -- PS-Simulink Converter6/LConn1
  Transform Sensor/RConn6 -- PS-Simulink Converter4/LConn1

== system ATRIAS_vnmc/atrias_system/Ground Contact/R Contact ==
  note: 3D Ground Interaction Model
  Env : Inport
  3D Contact : Subsystem
  Demux2 : Demux  Outputs=[1 3 3]
  External Force and Torque : sm_lib/Forces and Torques/External Force and Torque  ForceResolutionFrame=World  EnableForceX=off  EnableForceY=off  EnableForceZ=off  EnableForce=on  TorqueResolutionFrame=AttachedFrame  EnableTorqueX=off  EnableTorqueY=off  EnableTorqueZ=off  EnableTorque=off  BlockFunction=simmechanics.library.forces_torques.external_force_torque
  Mux1 : Mux  Inputs=3
  Mux2 : Mux  Inputs=3
  PS-Simulink Converter{1..6} (6 alike) : nesl_utility/PS-Simulink Converter  PhysicalDomain=network_engine_domain  SubClassName=ps_output  LeftPortType=input  RightPortType=output  PseudoPeriodic=off  Frequencies=[]  Unit=1  AffineConversion=off
  Simulink-PS Converter : nesl_utility/Simulink-PS Converter  PhysicalDomain=network_engine_domain  SubClassName=ps_input  LeftPortType=input  RightPortType=output  PseudoPeriodic=off  Frequencies=[]  NoiseDistribution=none  NoiseParameters=[]  Unit=1  AffineConversion=off  InputFiltering=off  SimscapeFilterOrder=1  InputFilterTimeConstant=0.001  UdotUserProvided=1
  Sum : Sum  Inputs=|+-
  Sum1 : Sum
  Transform Sensor : sm_lib/Frames and Transforms/Transform Sensor  MeasurementFrame=World  SenseAngle=off  SenseAxis=off  SenseAngle1=off  SenseAngle2=off  SenseAngle3=off  SenseQ=off  SenseR=off  SenseOmegaX=off  SenseOmegaY=off  SenseOmegaZ=off  SenseOmega1=off  SenseOmega2=off  SenseOmega3=off  SenseQDot=off  SenseRDot=off  SenseAlphaX=off  SenseAlphaY=off  SenseAlphaZ=off  SenseAlpha1=off  SenseAlpha2=off  SenseAlpha3=off  SenseQDDot=off  SenseRDDot=off  SenseX=on  SenseY=on  SenseZ=on  SenseRad=off  SenseAzim=off  SenseDist=off  SenseInc=off  SenseXDot=on  SenseYDot=on  SenseZDot=on  SenseRadDot=off  SenseAzimDot=off  SenseDistDot=off  SenseIncDot=off  SenseXDDot=off  SenseYDDot=off  SenseZDDot=off  SenseRadDDot=off  SenseAzimDDot=off  SenseDistDDot=off  SenseIncDDot=off  BlockFunction=simmechanics.library.frames_transforms.transform_sensor
  World Frame : sm_lib/Frames and Transforms/World Frame  BlockFunction=simmechanics.library.frames_transforms.world_frame
  contact? : simulink/Logic and Bit Operations/Compare To Zero  relop=<=  OutDataTypeStr=boolean
  y : Selector  InputPortWidth=3  Indices=2
  F : PMIOPort  Port=1  Side=Left
  RBallCnt : Outport
  GRF [N N N] : Outport  Port=2
  xyzFoot : Outport  Port=3
  wires:
  contact?/1 -> 3D Contact/Enable, RBallCnt/1  "cnt"
  Mux1/1 -> xyzFoot/1, 3D Contact/3(pVec [m m m]), y/1  "pos"
  Mux2/1 -> 3D Contact/4(vVec [m/s m/s m/s])
  Env/1 -> Demux2/1
  3D Contact/1(FnVec [N N N]) -> Sum1/1
  3D Contact/2(FtVec [N N N]) -> Sum1/2
  Sum1/1 -> Simulink-PS Converter/1, GRF [N N N]/1
  Sum/1 -> contact?/1
  y/1 -> Sum/1
  Demux2/1 -> Sum/2  "EnvHeight"
  Demux2/3 -> 3D Contact/2(nVec [m m m])  "Normal Vector nVec"
  Demux2/2 -> 3D Contact/1(RefPt [m m m])  "Reference Point RefPt"
  PS-Simulink Converter2/1 -> Mux1/1
  PS-Simulink Converter1/1 -> Mux1/2
  PS-Simulink Converter3/1 -> Mux1/3
  PS-Simulink Converter5/1 -> Mux2/1
  PS-Simulink Converter4/1 -> Mux2/2
  PS-Simulink Converter6/1 -> Mux2/3
  connections:
  External Force and Torque/LConn1 -- Simulink-PS Converter/RConn1
  External Force and Torque/RConn1 -- F/RConn1 -- Transform Sensor/RConn1
  World Frame/RConn1 -- Transform Sensor/LConn1
  PS-Simulink Converter2/LConn1 -- Transform Sensor/RConn2
  Transform Sensor/RConn3 -- PS-Simulink Converter1/LConn1
  Transform Sensor/RConn4 -- PS-Simulink Converter3/LConn1
  Transform Sensor/RConn5 -- PS-Simulink Converter5/LConn1
  Transform Sensor/RConn7 -- PS-Simulink Converter6/LConn1
  Transform Sensor/RConn6 -- PS-Simulink Converter4/LConn1

== system ATRIAS_vnmc/atrias_system/Ground Contact/roundTrack (LFoot) ==
  Cnt : Inport
  Gain : Gain  Gain=-1
  Gain1 : Gain  Gain=-1
  Ground H1 : Interpolation_n-D  NumberOfTableDimensions=1  Table=v_plateH
      settings: InputPortMap=u0,u1
  Ground Slope : Interpolation_n-D  NumberOfTableDimensions=1  Table=v_plateS  InterpMethod=Flat
      settings: InputPortMap=u0,u1
  Mux : Mux  Inputs=7
  Prelookup : PreLookup  BreakpointsData=v_plateYaw  ExtrapMethod=Linear
  Product : Product
  Product1 : Product
  Selector1 : Selector  InputPortWidth=3  Indices=[1 3]
  Selector22 : Selector  InputPortWidth=3  Indices=3
  Selector23 : Selector  InputPortWidth=3
  Trigonometric Function1 : Trigonometry
  Trigonometric Function2 : Trigonometry  Operator=cos
  Trigonometric Function3 : Trigonometry
  Trigonometric Function4 : Trigonometry  Operator=cos
  track yaw : Subsystem
  Env : Outport
  wires:
  Selector22/1 -> Mux/4
  Prelookup/1 -> Ground H1/1, Ground Slope/1
  Ground Slope/1 -> Trigonometric Function2/1, Trigonometric Function1/1
  Trigonometric Function2/1 -> Mux/6  "nv"
  Trigonometric Function1/1 -> Gain/1
  Prelookup/2 -> Ground H1/2, Ground Slope/2
  Selector23/1 -> Mux/2
  Selector1/1 -> track yaw/1(xz)
  track yaw/1(yaw) -> Trigonometric Function4/1, Trigonometric Function3/1, Prelookup/1
  Gain/1 -> Product/1, Product1/1  "nt"
  Trigonometric Function3/1 -> Gain1/1
  Trigonometric Function4/1 -> Product/2
  Product/1 -> Mux/5  "nx"
  Product1/1 -> Mux/7  "nz"
  Gain1/1 -> Product1/2
  Mux/1 -> Env/1
  Ground H1/1 -> Mux/3, Mux/1  "EnvHeight"
  Cnt/1 -> Selector1/1, Selector22/1, Selector23/1

== system ATRIAS_vnmc/atrias_system/Ground Contact/roundTrack (RFoot) ==
  Cnt : Inport
  Gain : Gain  Gain=-1
  Gain1 : Gain  Gain=-1
  Ground H1 : Interpolation_n-D  NumberOfTableDimensions=1  Table=v_plateH
      settings: InputPortMap=u0,u1
  Ground Slope : Interpolation_n-D  NumberOfTableDimensions=1  Table=v_plateS  InterpMethod=Flat
      settings: InputPortMap=u0,u1
  Mux : Mux  Inputs=7
  Prelookup : PreLookup  BreakpointsData=v_plateYaw  ExtrapMethod=Linear
  Product : Product
  Product1 : Product
  Selector1 : Selector  InputPortWidth=3  Indices=[1 3]
  Selector22 : Selector  InputPortWidth=3  Indices=3
  Selector23 : Selector  InputPortWidth=3
  Trigonometric Function1 : Trigonometry
  Trigonometric Function2 : Trigonometry  Operator=cos
  Trigonometric Function3 : Trigonometry
  Trigonometric Function4 : Trigonometry  Operator=cos
  track yaw : Subsystem
  Env : Outport
  wires:
  Selector22/1 -> Mux/4
  Prelookup/1 -> Ground H1/1, Ground Slope/1
  Ground Slope/1 -> Trigonometric Function2/1, Trigonometric Function1/1
  Trigonometric Function2/1 -> Mux/6  "nv"
  Trigonometric Function1/1 -> Gain/1
  Prelookup/2 -> Ground H1/2, Ground Slope/2
  Selector23/1 -> Mux/2
  Selector1/1 -> track yaw/1(xz)
  track yaw/1(yaw) -> Trigonometric Function4/1, Trigonometric Function3/1, Prelookup/1
  Gain/1 -> Product/1, Product1/1  "nt"
  Trigonometric Function3/1 -> Gain1/1
  Trigonometric Function4/1 -> Product/2
  Product/1 -> Mux/5  "nx"
  Product1/1 -> Mux/7  "nz"
  Gain1/1 -> Product1/2
  Mux/1 -> Env/1
  Ground H1/1 -> Mux/3, Mux/1  "EnvHeight"
  Cnt/1 -> Selector1/1, Selector22/1, Selector23/1
